simulink model "e8_t1"  (R2024b)
settings: Solver=VariableStepAuto  StartTime=0.0  StopTime=10.0  RelTol=1e-3

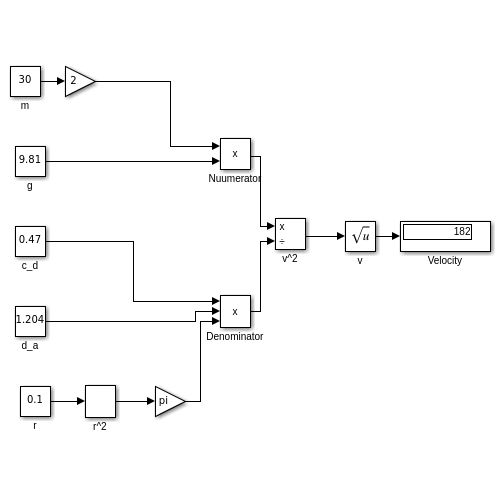
[thumbnail: Simulink's stored preview of the top-level diagram]
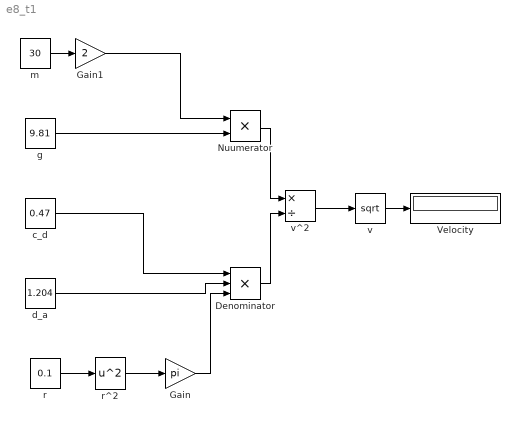
== system e8_t1 ==
  Denominator : Product  Inputs=3
  Gain : Gain  Gain=pi
  Gain1 : Gain  Gain=2
  Nuumerator : Product
  Velocity : Display
  c_d : Constant  Value=0.47
  d_a : Constant  Value=1.204
  g : Constant  Value=9.81
  m : Constant  Value=30
  r : Constant  Value=0.1
  r^2 : Math  Operator=square
  v : Sqrt
  v^2 : Product  Inputs=*/
  wires:
  r/1 -> r^2/1
  r^2/1 -> Gain/1
  Gain/1 -> Denominator/3
  d_a/1 -> Denominator/2
  c_d/1 -> Denominator/1
  m/1 -> Gain1/1
  g/1 -> Nuumerator/2
  Gain1/1 -> Nuumerator/1
  Nuumerator/1 -> v^2/1
  Denominator/1 -> v^2/2
  v^2/1 -> v/1
  v/1 -> Velocity/1
